simulink model "Plant_1_3"  (R2024b)
settings: Solver=VariableStepAuto  StartTime=0.0  StopTime=2  RelTol=1e-3
PreLoadFcn:
  | addpath ref_source\2s\
values from neighbouring files (symbols this model uses):
  A = [ 0   1   0 ... (first row only)    [state_feedback_2.m]
  B = [ 0 ... (first row only)    [state_feedback_2.m]
undefined symbols (not defined in the file or in its folder): L1, L2, plnt1_2_kd_th1, plnt1_2_kd_th2, plnt1_2_ki_th1, plnt1_2_ki_th2, plnt1_2_kp_th1, plnt1_2_kp_th2, plnt1_2_N_th1, plnt1_2_N_th2
libraries: slpidlib x2
settings Model: Creator=Sez26  LastModifiedBy=Sez26

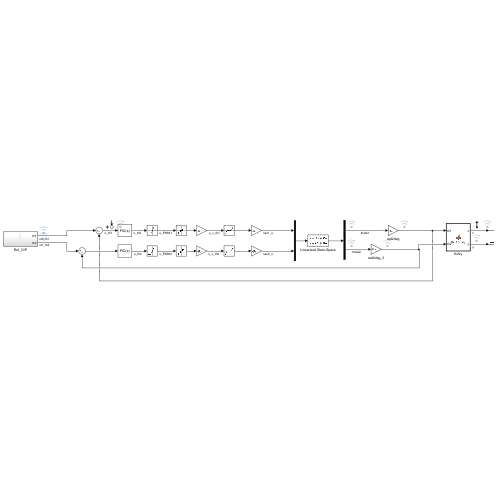
[thumbnail: Simulink's stored preview of the top-level diagram]
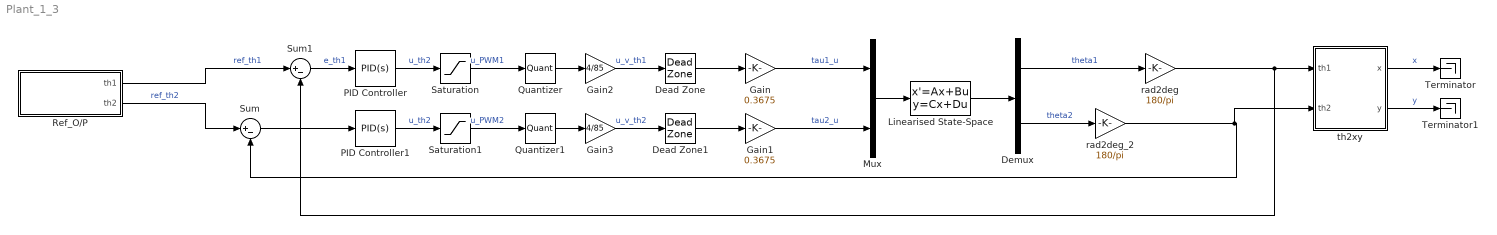
== system Plant_1_3 ==
  Dead Zone : DeadZone  LowerValue=-2.1  UpperValue=2.1
  Dead Zone1 : DeadZone  LowerValue=-2.1  UpperValue=2.1
  Demux : Demux  Outputs=2
  Gain : Gain  Gain=0.3675
  Gain1 : Gain  Gain=0.3675
  Gain2 : Gain  Gain=4/85
  Gain3 : Gain  Gain=4/85
  Linearised State-Space : StateSpace  A=A  B=B  C=[1 0 0 0; 0 1 0 0]  D=[0 0; 0 0]  InitialCondition=0
  Mux : Mux  Inputs=2
  PID Controller : slpidlib/PID Controller  Controller=PID  Form=Parallel  TimeDomain=Continuous-time  UseExternalTs=off  SampleTime=-1  IntegratorMethod=Forward Euler  FilterMethod=Forward Euler  ControllerParametersSource=internal  P=plnt1_2_kp_th1  I=plnt1_2_ki_th1  UseKiTs=off  D=plnt1_2_kd_th1  UseExternalDerivativeSource=off  N=plnt1_2_N_th1  UseFilter=on  TunerSelectOption=Transfer Function Based (PID Tuner App)  InitialConditionSource=internal  InitialConditionForIntegrator=0  InitialConditionForFilter=0  DifferentiatorICPrevScaledInput=0  ExternalReset=none  TrackingMode=off  Kt=1  LimitOutput=off  SatLimitsSource=internal  UpperSaturationLimit=inf  LowerSaturationLimit=-inf  LinearizeAsGain=on  AntiWindupMode=none  Kb=1  LimitIntegrator=off  UpperIntegratorSaturationLimit=inf  LowerIntegratorSaturationLimit=-inf  POutMin=[]  POutMax=[]  IOutMin=[]  IOutMax=[]  DOutMin=[]  DOutMax=[]  NOutMin=[]  NOutMax=[]  SumOutMin=[]  SumOutMax=[]  SaturationOutMin=[]  SaturationOutMax=[]  PParamMin=[]  PParamMax=[]  IParamMin=[]  IParamMax=[]  DParamMin=[]  DParamMax=[]  NParamMin=[]  NParamMax=[]  KbParamMin=[]  KbParamMax=[]  KtParamMin=[]  KtParamMax=[]  KbOutMin=[]  KbOutMax=[]  KtOutMin=[]  KtOutMax=[]  IntegratorOutMin=[]  IntegratorOutMax=[]  FilterOutMin=[]  FilterOutMax=[]  SumI1OutMin=[]  SumI1OutMax=[]  SumI2OutMin=[]  SumI2OutMax=[]  SumI3OutMin=[]  SumI3OutMax=[]  SumI4OutMin=[]  SumI4OutMax=[]  SumDOutMin=[]  SumDOutMax=[]  DifferentiatorOutMin=[]  DifferentiatorOutMax=[]  FilterDiffOutCoefMin=[]  FilterDiffOutCoefMax=[]  ReciprocalOutMin=[]  ReciprocalOutMax=[]  SumDenOutMin=[]  SumDenOutMax=[]  SumNumOutMin=[]  SumNumOutMax=[]  DivideOutMin=[]  DivideOutMax=[]  UdiffTsProdOutMin=[]  UdiffTsProdOutMax=[]  NTsProdOutMin=[]  NTsProdOutMax=[]  UintegralTsProdOutMin=[]  UintegralTsProdOutMax=[]  UngainTsProdOutMin=[]  UngainTsProdOutMax=[]  ClampingZeroOutDataTypeStr=Inherit: Inherit via back propagation  ClampingZeroOutMin=[]  ClampingZeroOutMax=[]  FilterDenConstantOutDataTypeStr=Inherit: Inherit via back propagation  FilterDenConstantOutMin=[]  FilterDenConstantOutMax=[]  PCopyOutDataTypeStr=Inherit: Inherit via back propagation  PCopyOutMin=[]  PCopyOutMax=[]  NCopyOutDataTypeStr=Inherit: Inherit via back propagation  NCopyOutMin=[]  NCopyOutMax=[]  IntegratorContinuousStateAttributes=''  IntegratorStateMustResolveToSignalObject=off  IntegratorRTWStateStorageClass=Auto  FilterContinuousStateAttributes=''  FilterStateMustResolveToSignalObject=off  FilterRTWStateStorageClass=Auto  ParallelPVariant=InternalParameters  IdealPVariant=Disabled  IVariant=InternalParameters  DVariant=InternalParameters  IntegratorVariant=Continuous  SatVariant=Disabled  AWVariant=Passthrough  PCopyVariant=Disabled  TRVariant=Disabled  FdbkBlocksVariant=Forward  IdealPFdbkVariant=Disabled  SatFdbkVariant=Disabled  DerivativeFilterVariant=ContFilter  NVariant=InternalParameters  NCopyVariant=Disabled  FilterICVariant=InternalICsFilter  IntegratorICVariant=InternalICs  ExternalResetVariant=Disabled  TRSumVariant=Passthrough  SumFdbkVariant=Disabled  SumVariant=Sum_PID  TsampFilterVariant=InternalTs  TsampNgainVariant=Passthrough  TsampIntegralVariant=Disabled_SignalSpec  ExternalSaturationOutDataTypeStr=Inherit: Same as second input  DerivativeSourceVariant=ErrorSignal  PreIntVariant=InternalPreInt
  PID Controller1 : slpidlib/PID Controller  Controller=PID  Form=Parallel  TimeDomain=Continuous-time  UseExternalTs=off  SampleTime=-1  IntegratorMethod=Forward Euler  FilterMethod=Forward Euler  ControllerParametersSource=internal  P=plnt1_2_kp_th2  I=plnt1_2_ki_th2  UseKiTs=off  D=plnt1_2_kd_th2  UseExternalDerivativeSource=off  N=plnt1_2_N_th2  UseFilter=on  TunerSelectOption=Transfer Function Based (PID Tuner App)  InitialConditionSource=internal  InitialConditionForIntegrator=0  InitialConditionForFilter=0  DifferentiatorICPrevScaledInput=0  ExternalReset=none  TrackingMode=off  Kt=1  LimitOutput=off  SatLimitsSource=internal  UpperSaturationLimit=inf  LowerSaturationLimit=-inf  LinearizeAsGain=on  AntiWindupMode=none  Kb=1  LimitIntegrator=off  UpperIntegratorSaturationLimit=inf  LowerIntegratorSaturationLimit=-inf  POutMin=[]  POutMax=[]  IOutMin=[]  IOutMax=[]  DOutMin=[]  DOutMax=[]  NOutMin=[]  NOutMax=[]  SumOutMin=[]  SumOutMax=[]  SaturationOutMin=[]  SaturationOutMax=[]  PParamMin=[]  PParamMax=[]  IParamMin=[]  IParamMax=[]  DParamMin=[]  DParamMax=[]  NParamMin=[]  NParamMax=[]  KbParamMin=[]  KbParamMax=[]  KtParamMin=[]  KtParamMax=[]  KbOutMin=[]  KbOutMax=[]  KtOutMin=[]  KtOutMax=[]  IntegratorOutMin=[]  IntegratorOutMax=[]  FilterOutMin=[]  FilterOutMax=[]  SumI1OutMin=[]  SumI1OutMax=[]  SumI2OutMin=[]  SumI2OutMax=[]  SumI3OutMin=[]  SumI3OutMax=[]  SumI4OutMin=[]  SumI4OutMax=[]  SumDOutMin=[]  SumDOutMax=[]  DifferentiatorOutMin=[]  DifferentiatorOutMax=[]  FilterDiffOutCoefMin=[]  FilterDiffOutCoefMax=[]  ReciprocalOutMin=[]  ReciprocalOutMax=[]  SumDenOutMin=[]  SumDenOutMax=[]  SumNumOutMin=[]  SumNumOutMax=[]  DivideOutMin=[]  DivideOutMax=[]  UdiffTsProdOutMin=[]  UdiffTsProdOutMax=[]  NTsProdOutMin=[]  NTsProdOutMax=[]  UintegralTsProdOutMin=[]  UintegralTsProdOutMax=[]  UngainTsProdOutMin=[]  UngainTsProdOutMax=[]  ClampingZeroOutDataTypeStr=Inherit: Inherit via back propagation  ClampingZeroOutMin=[]  ClampingZeroOutMax=[]  FilterDenConstantOutDataTypeStr=Inherit: Inherit via back propagation  FilterDenConstantOutMin=[]  FilterDenConstantOutMax=[]  PCopyOutDataTypeStr=Inherit: Inherit via back propagation  PCopyOutMin=[]  PCopyOutMax=[]  NCopyOutDataTypeStr=Inherit: Inherit via back propagation  NCopyOutMin=[]  NCopyOutMax=[]  IntegratorContinuousStateAttributes=''  IntegratorStateMustResolveToSignalObject=off  IntegratorRTWStateStorageClass=Auto  FilterContinuousStateAttributes=''  FilterStateMustResolveToSignalObject=off  FilterRTWStateStorageClass=Auto  ParallelPVariant=InternalParameters  IdealPVariant=Disabled  IVariant=InternalParameters  DVariant=InternalParameters  IntegratorVariant=Continuous  SatVariant=Disabled  AWVariant=Passthrough  PCopyVariant=Disabled  TRVariant=Disabled  FdbkBlocksVariant=Forward  IdealPFdbkVariant=Disabled  SatFdbkVariant=Disabled  DerivativeFilterVariant=ContFilter  NVariant=InternalParameters  NCopyVariant=Disabled  FilterICVariant=InternalICsFilter  IntegratorICVariant=InternalICs  ExternalResetVariant=Disabled  TRSumVariant=Passthrough  SumFdbkVariant=Disabled  SumVariant=Sum_PID  TsampFilterVariant=InternalTs  TsampNgainVariant=Passthrough  TsampIntegralVariant=Disabled_SignalSpec  ExternalSaturationOutDataTypeStr=Inherit: Same as second input  DerivativeSourceVariant=ErrorSignal  PreIntVariant=InternalPreInt
  Quantizer : Quantizer  QuantizationInterval=1
  Quantizer1 : Quantizer  QuantizationInterval=1
  Ref_O/P : Subsystem
  Saturation : Saturate  UpperLimit=255  LowerLimit=-255
  Saturation1 : Saturate  UpperLimit=255  LowerLimit=-255
  Sum : Sum  Inputs=|+-
  Sum1 : Sum  Inputs=|+-
  Terminator : Terminator
  Terminator1 : Terminator
  rad2deg : Gain  Gain=180/pi
  rad2deg_2 : Gain  Gain=180/pi
  th2xy : MATLAB Function  TreatAsAtomicUnit=on
  wires:
  Linearised State-Space/1 -> Demux/1
  Demux/1 -> rad2deg/1  "theta1"
  Demux/2 -> rad2deg_2/1  "theta2"
  Sum/1 -> PID Controller1/1
  Sum1/1 -> PID Controller/1  "e_th1"
  Gain3/1 -> Dead Zone1/1  "u_v_th2"
  PID Controller/1 -> Saturation/1  "u_th2"
  Quantizer1/1 -> Gain3/1
  PID Controller1/1 -> Saturation1/1  "u_th2"
  Saturation/1 -> Quantizer/1  "u_PWM1"
  Dead Zone/1 -> Gain/1
  Quantizer/1 -> Gain2/1
  Gain2/1 -> Dead Zone/1  "u_v_th1"
  Dead Zone1/1 -> Gain1/1
  Saturation1/1 -> Quantizer1/1  "u_PWM2"
  Ref_O/P/1(th1) -> Sum1/1  "ref_th1"
  Ref_O/P/2(th2) -> Sum/1  "ref_th2"
  Mux/1 -> Linearised State-Space/1
  Gain/1 -> Mux/1  "tau1_u"
  Gain1/1 -> Mux/2  "tau2_u"
  rad2deg/1 -> th2xy/1(th1), Sum1/2
  rad2deg_2/1 -> th2xy/2(th2), Sum/2
  th2xy/1(x) -> Terminator/1  "x"
  th2xy/2(y) -> Terminator1/1  "y"

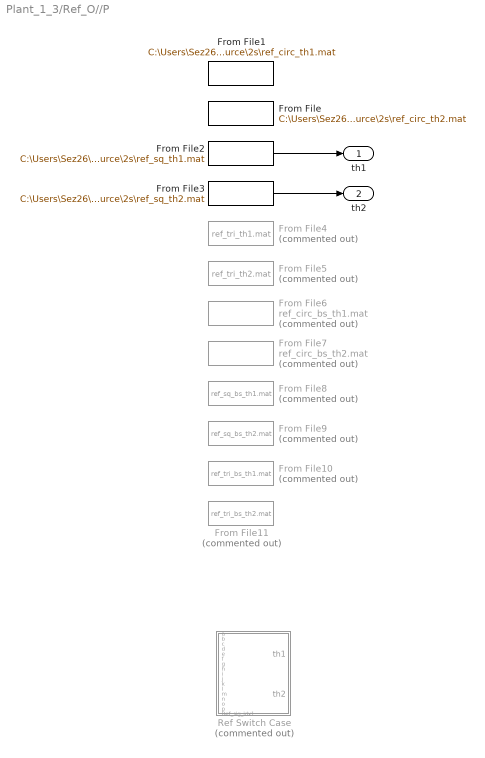
== system Plant_1_3/Ref_O//P ==
  From File : FromFile  FileName=C:\Users\Sez26\Documents\Arduino\MVNLC\control\Uni2024_MVNLC\Simulink_Simulation\ref_source\2s\ref_circ_th2.mat  SampleTime=0
  From File1 : FromFile  FileName=C:\Users\Sez26\Documents\Arduino\MVNLC\control\Uni2024_MVNLC\Simulink_Simulation\ref_source\2s\ref_circ_th1.mat  SampleTime=0
  From File10 : FromFile  Commented=on  FileName=ref_tri_bs_th1.mat  SampleTime=0
  From File11 : FromFile  Commented=on  FileName=ref_tri_bs_th2.mat  SampleTime=0
  From File2 : FromFile  FileName=C:\Users\Sez26\Documents\Arduino\MVNLC\control\Uni2024_MVNLC\Simulink_Simulation\ref_source\2s\ref_sq_th1.mat  SampleTime=0
  From File3 : FromFile  FileName=C:\Users\Sez26\Documents\Arduino\MVNLC\control\Uni2024_MVNLC\Simulink_Simulation\ref_source\2s\ref_sq_th2.mat  SampleTime=0
  From File4 : FromFile  Commented=on  FileName=ref_tri_th1.mat  SampleTime=0
  From File5 : FromFile  Commented=on  FileName=ref_tri_th2.mat  SampleTime=0
  From File6 : FromFile  Commented=on  FileName=ref_circ_bs_th1.mat  SampleTime=0
  From File7 : FromFile  Commented=on  FileName=ref_circ_bs_th2.mat  SampleTime=0
  From File8 : FromFile  Commented=on  FileName=ref_sq_bs_th1.mat  SampleTime=0
  From File9 : FromFile  Commented=on  FileName=ref_sq_bs_th2.mat  SampleTime=0
  Ref Switch Case : MATLAB Function  Commented=on  TreatAsAtomicUnit=on
  th1 : Outport
  th2 : Outport  Port=2
  wires:
  From File3/1 -> th2/1
  From File2/1 -> th1/1

== matlab function Plant_1_3/Ref_O//P/Ref Switch Case ==
  data: Ref_sig_idx parameter; a input; b input; c input; d input; e input; f input; g input; h input; i input; j input; k input; l input; m input; n input; o input; p input; Ref_sig_idx1 input; th1 output; th2 output
function [th1, th2] = ref_switch(Ref_sig_idx, a, b, c, d, e, f, g, h, i, j, k, l, m, n, o, p, Ref_sig_idx1)
    if Ref_sig_idx == 0
        % circ base
        th1 = a;
        th2 = b;
    elseif Ref_sig_idx == 1
        % sq base
        th1 = c;
        th2 = d;
    elseif Ref_sig_idx == 2
        % tri base
        th1 = e;
        th2 = f;
    end
    if Ref_sig_idx == 3
        % circ b spline
        th1 = g;
        th2 = h;
    elseif Ref_sig_idx == 4
        % sq b spline
        th1 = i;
        th2 = j;
    elseif Ref_sig_idx == 5
        % tri b spline
        th1 = k;
        th2 = l;
    end
    if Ref_sig_idx == 6
        % sq corner sf
        th1 = m;
        th2 = n;
    elseif Ref_sig_idx == 7
        % tri corner sf
        th1 = o;
        th2 = p;
    else
        % invalid reference choice
        disp('Error invalid reference choice')
        th1 = 0;
        th2 = 0;
    end

== matlab function Plant_1_3/th2xy ==
  data: x output; th1 input; y output; th2 input; L1 parameter; L2 parameter
function [x,y] = th_to_xy(th1, th2, L1, L2)
    x = L1*cos(deg2rad(th1)) + L2*cos(deg2rad(th2));
    y = L1*sin(deg2rad(th1)) + L2*sin(deg2rad(th2));
